simulink model "Manipulator_Dynamics_testing"  (R2019b)
settings: Solver=ode1  StartTime=0.0  StopTime=10  FixedStep=1e-3  RelTol=1e-3  AbsTol=1e-3
InitFcn:
  | parameters
values from neighbouring files (symbols this model uses):
  a = 140/1000    (= 0.14)    [parameters.m]
  d = 23/2000    (= 0.0115)    [parameters.m]
  eta = 0.39    [parameters.m]
  g = 9.81    [parameters.m]
  l_link = a-2*d    (= 0.117)    [parameters.m]
  m = 0.2    [parameters.m]
  mu_cable = 0.17    [parameters.m]
  r = 20.5/1000    (= 0.0205)    [parameters.m]
  r_drum = 0.042    [parameters.m]
libraries: simulink x27, dspindex x18, dspinverses x1
(part 1 of 5)
settings Model: Creator=arund  LastModifiedBy=arund
settings SolverCC: MaxConsecutiveMinStep=10
settings DataIOCC: SaveState=on

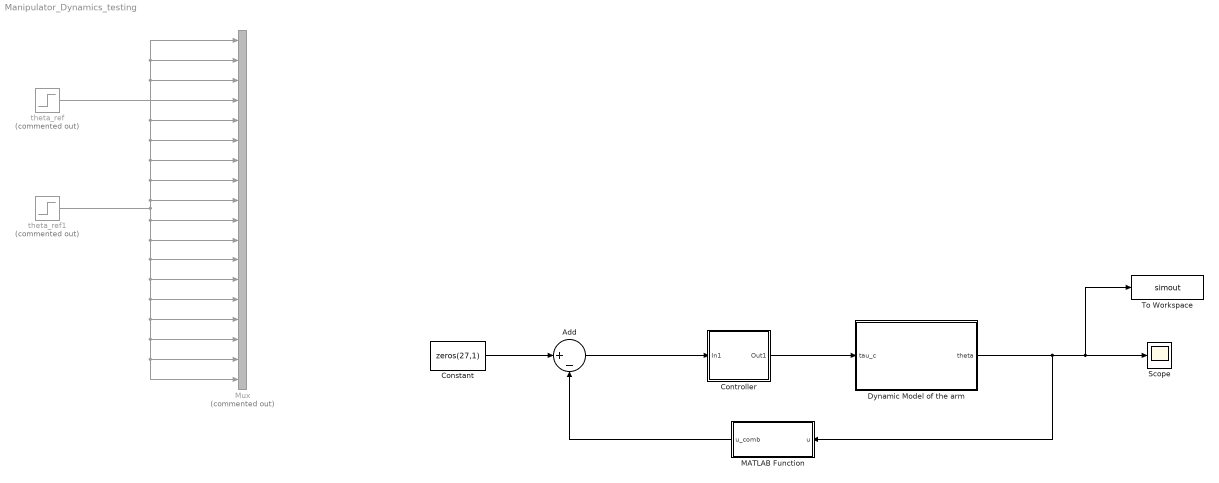
== system Manipulator_Dynamics_testing ==
  Add : Sum  Inputs=|+-
  Constant : Constant  Value=zeros(27,1)
  Controller : Subsystem
  Dynamic Model of the arm : Subsystem
  MATLAB Function : MATLAB Function  TreatAsAtomicUnit=on
  Mux : Mux  Commented=on  Inputs=18
  Scope : Scope
  To Workspace : ToWorkspace  VariableName=simout  SampleTime=-1
  theta_ref : Step  Commented=on  SampleTime=0
  theta_ref1 : Step  Commented=on  After=0  SampleTime=0
  wires:
  Dynamic Model of the arm/1(theta) -> To Workspace/1, Scope/1, MATLAB Function/1(u)
  theta_ref/1 -> Mux/4
  theta_ref1/1 -> Mux/6, Mux/5, Mux/3, Mux/2, Mux/1, Mux/7, Mux/8, Mux/9, Mux/14, Mux/15, Mux/16, Mux/17, Mux/18, Mux/13, Mux/12, Mux/11, Mux/10
  Constant/1 -> Add/1
  MATLAB Function/1(u_comb) -> Add/2
  Add/1 -> Controller/1(In1)
  Controller/1(Out1) -> Dynamic Model of the arm/1(tau_c)

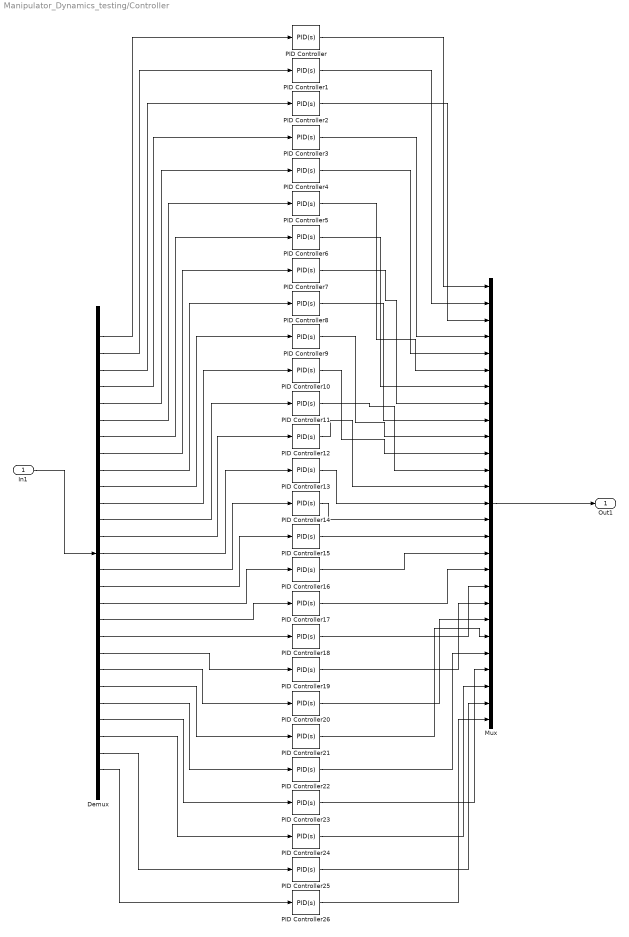
== system Manipulator_Dynamics_testing/Controller ==
  In1 : Inport
  Demux : Demux  Outputs=27
  Mux : Mux  Inputs=27
  PID Controller{,1..23} (24 alike) : simulink/Continuous/PID Controller  Controller=PID  Form=Parallel  TimeDomain=Continuous-time  SampleTime=-1  IntegratorMethod=Forward Euler  FilterMethod=Forward Euler  ControllerParametersSource=internal  P=0  I=0  D=0  UseFilter=on  N=100  TunerSelectOption=Transfer Function Based (PID Tuner App)  InitialConditionSource=internal  InitialConditionForIntegrator=0  InitialConditionForFilter=0  DifferentiatorICPrevScaledInput=0  ExternalReset=none  TrackingMode=off  Kt=1  LimitOutput=off  UpperSaturationLimit=inf  LowerSaturationLimit=-inf  LinearizeAsGain=on  AntiWindupMode=none  Kb=1  POutMin=[]  POutMax=[]  IOutMin=[]  IOutMax=[]  DOutMin=[]  DOutMax=[]  NOutMin=[]  NOutMax=[]  SumOutMin=[]  SumOutMax=[]  SaturationOutMin=[]  SaturationOutMax=[]  PParamMin=[]  PParamMax=[]  IParamMin=[]  IParamMax=[]  DParamMin=[]  DParamMax=[]  NParamMin=[]  NParamMax=[]  KbParamMin=[]  KbParamMax=[]  KtParamMin=[]  KtParamMax=[]  KbOutMin=[]  KbOutMax=[]  KtOutMin=[]  KtOutMax=[]  IntegratorOutMin=[]  IntegratorOutMax=[]  FilterOutMin=[]  FilterOutMax=[]  SumI1OutMin=[]  SumI1OutMax=[]  SumI2OutMin=[]  SumI2OutMax=[]  SumI3OutMin=[]  SumI3OutMax=[]  SumI4OutMin=[]  SumI4OutMax=[]  SumDOutMin=[]  SumDOutMax=[]  DifferentiatorOutMin=[]  DifferentiatorOutMax=[]  FilterDiffOutCoefMin=[]  FilterDiffOutCoefMax=[]  ReciprocalOutMin=[]  ReciprocalOutMax=[]  SumDenOutMin=[]  SumDenOutMax=[]  SumNumOutMin=[]  SumNumOutMax=[]  DivideOutMin=[]  DivideOutMax=[]  IntegratorContinuousStateAttributes=''  IntegratorStateMustResolveToSignalObject=off  IntegratorRTWStateStorageClass=Auto  FilterContinuousStateAttributes=''  FilterStateMustResolveToSignalObject=off  FilterRTWStateStorageClass=Auto  ParallelPVariant=InternalParameters  IdealPVariant=Disabled  IVariant=InternalParameters  DVariant=InternalParameters  IntegratorVariant=Continuous  SatVariant=Disabled  AWVariant=Passthrough  PCopyVariant=Disabled  TRVariant=Disabled  FdbkBlocksVariant=Forward  IdealPFdbkVariant=Disabled  SatFdbkVariant=Disabled  DerivativeFilterVariant=ContFilter  NVariant=InternalParameters  NCopyVariant=Disabled  FilterICVariant=InternalICsFilter  IntegratorICVariant=InternalICs  ExternalResetVariant=Disabled  TRSumVariant=Passthrough  SumFdbkVariant=Disabled  SumVariant=Sum_PID
  PID Controller24 : simulink/Continuous/PID Controller  Controller=PID  Form=Parallel  TimeDomain=Continuous-time  SampleTime=-1  IntegratorMethod=Forward Euler  FilterMethod=Forward Euler  ControllerParametersSource=internal  P=10  I=0  D=10  UseFilter=on  N=100  TunerSelectOption=Transfer Function Based (PID Tuner App)  InitialConditionSource=internal  InitialConditionForIntegrator=0  InitialConditionForFilter=0  DifferentiatorICPrevScaledInput=0  ExternalReset=none  TrackingMode=off  Kt=1  LimitOutput=off  UpperSaturationLimit=inf  LowerSaturationLimit=-inf  LinearizeAsGain=on  AntiWindupMode=none  Kb=1  POutMin=[]  POutMax=[]  IOutMin=[]  IOutMax=[]  DOutMin=[]  DOutMax=[]  NOutMin=[]  NOutMax=[]  SumOutMin=[]  SumOutMax=[]  SaturationOutMin=[]  SaturationOutMax=[]  PParamMin=[]  PParamMax=[]  IParamMin=[]  IParamMax=[]  DParamMin=[]  DParamMax=[]  NParamMin=[]  NParamMax=[]  KbParamMin=[]  KbParamMax=[]  KtParamMin=[]  KtParamMax=[]  KbOutMin=[]  KbOutMax=[]  KtOutMin=[]  KtOutMax=[]  IntegratorOutMin=[]  IntegratorOutMax=[]  FilterOutMin=[]  FilterOutMax=[]  SumI1OutMin=[]  SumI1OutMax=[]  SumI2OutMin=[]  SumI2OutMax=[]  SumI3OutMin=[]  SumI3OutMax=[]  SumI4OutMin=[]  SumI4OutMax=[]  SumDOutMin=[]  SumDOutMax=[]  DifferentiatorOutMin=[]  DifferentiatorOutMax=[]  FilterDiffOutCoefMin=[]  FilterDiffOutCoefMax=[]  ReciprocalOutMin=[]  ReciprocalOutMax=[]  SumDenOutMin=[]  SumDenOutMax=[]  SumNumOutMin=[]  SumNumOutMax=[]  DivideOutMin=[]  DivideOutMax=[]  IntegratorContinuousStateAttributes=''  IntegratorStateMustResolveToSignalObject=off  IntegratorRTWStateStorageClass=Auto  FilterContinuousStateAttributes=''  FilterStateMustResolveToSignalObject=off  FilterRTWStateStorageClass=Auto  ParallelPVariant=InternalParameters  IdealPVariant=Disabled  IVariant=InternalParameters  DVariant=InternalParameters  IntegratorVariant=Continuous  SatVariant=Disabled  AWVariant=Passthrough  PCopyVariant=Disabled  TRVariant=Disabled  FdbkBlocksVariant=Forward  IdealPFdbkVariant=Disabled  SatFdbkVariant=Disabled  DerivativeFilterVariant=ContFilter  NVariant=InternalParameters  NCopyVariant=Disabled  FilterICVariant=InternalICsFilter  IntegratorICVariant=InternalICs  ExternalResetVariant=Disabled  TRSumVariant=Passthrough  SumFdbkVariant=Disabled  SumVariant=Sum_PID
  PID Controller25 : simulink/Continuous/PID Controller  Controller=PID  Form=Parallel  TimeDomain=Continuous-time  SampleTime=-1  IntegratorMethod=Forward Euler  FilterMethod=Forward Euler  ControllerParametersSource=internal  P=10  I=0  D=10  UseFilter=on  N=100  TunerSelectOption=Transfer Function Based (PID Tuner App)  InitialConditionSource=internal  InitialConditionForIntegrator=0  InitialConditionForFilter=0  DifferentiatorICPrevScaledInput=0  ExternalReset=none  TrackingMode=off  Kt=1  LimitOutput=off  UpperSaturationLimit=inf  LowerSaturationLimit=-inf  LinearizeAsGain=on  AntiWindupMode=none  Kb=1  POutMin=[]  POutMax=[]  IOutMin=[]  IOutMax=[]  DOutMin=[]  DOutMax=[]  NOutMin=[]  NOutMax=[]  SumOutMin=[]  SumOutMax=[]  SaturationOutMin=[]  SaturationOutMax=[]  PParamMin=[]  PParamMax=[]  IParamMin=[]  IParamMax=[]  DParamMin=[]  DParamMax=[]  NParamMin=[]  NParamMax=[]  KbParamMin=[]  KbParamMax=[]  KtParamMin=[]  KtParamMax=[]  KbOutMin=[]  KbOutMax=[]  KtOutMin=[]  KtOutMax=[]  IntegratorOutMin=[]  IntegratorOutMax=[]  FilterOutMin=[]  FilterOutMax=[]  SumI1OutMin=[]  SumI1OutMax=[]  SumI2OutMin=[]  SumI2OutMax=[]  SumI3OutMin=[]  SumI3OutMax=[]  SumI4OutMin=[]  SumI4OutMax=[]  SumDOutMin=[]  SumDOutMax=[]  DifferentiatorOutMin=[]  DifferentiatorOutMax=[]  FilterDiffOutCoefMin=[]  FilterDiffOutCoefMax=[]  ReciprocalOutMin=[]  ReciprocalOutMax=[]  SumDenOutMin=[]  SumDenOutMax=[]  SumNumOutMin=[]  SumNumOutMax=[]  DivideOutMin=[]  DivideOutMax=[]  IntegratorContinuousStateAttributes=''  IntegratorStateMustResolveToSignalObject=off  IntegratorRTWStateStorageClass=Auto  FilterContinuousStateAttributes=''  FilterStateMustResolveToSignalObject=off  FilterRTWStateStorageClass=Auto  ParallelPVariant=InternalParameters  IdealPVariant=Disabled  IVariant=InternalParameters  DVariant=InternalParameters  IntegratorVariant=Continuous  SatVariant=Disabled  AWVariant=Passthrough  PCopyVariant=Disabled  TRVariant=Disabled  FdbkBlocksVariant=Forward  IdealPFdbkVariant=Disabled  SatFdbkVariant=Disabled  DerivativeFilterVariant=ContFilter  NVariant=InternalParameters  NCopyVariant=Disabled  FilterICVariant=InternalICsFilter  IntegratorICVariant=InternalICs  ExternalResetVariant=Disabled  TRSumVariant=Passthrough  SumFdbkVariant=Disabled  SumVariant=Sum_PID
  PID Controller26 : simulink/Continuous/PID Controller  Controller=PID  Form=Parallel  TimeDomain=Continuous-time  SampleTime=-1  IntegratorMethod=Forward Euler  FilterMethod=Forward Euler  ControllerParametersSource=internal  P=10  I=0  D=10  UseFilter=on  N=100  TunerSelectOption=Transfer Function Based (PID Tuner App)  InitialConditionSource=internal  InitialConditionForIntegrator=0  InitialConditionForFilter=0  DifferentiatorICPrevScaledInput=0  ExternalReset=none  TrackingMode=off  Kt=1  LimitOutput=off  UpperSaturationLimit=inf  LowerSaturationLimit=-inf  LinearizeAsGain=on  AntiWindupMode=none  Kb=1  POutMin=[]  POutMax=[]  IOutMin=[]  IOutMax=[]  DOutMin=[]  DOutMax=[]  NOutMin=[]  NOutMax=[]  SumOutMin=[]  SumOutMax=[]  SaturationOutMin=[]  SaturationOutMax=[]  PParamMin=[]  PParamMax=[]  IParamMin=[]  IParamMax=[]  DParamMin=[]  DParamMax=[]  NParamMin=[]  NParamMax=[]  KbParamMin=[]  KbParamMax=[]  KtParamMin=[]  KtParamMax=[]  KbOutMin=[]  KbOutMax=[]  KtOutMin=[]  KtOutMax=[]  IntegratorOutMin=[]  IntegratorOutMax=[]  FilterOutMin=[]  FilterOutMax=[]  SumI1OutMin=[]  SumI1OutMax=[]  SumI2OutMin=[]  SumI2OutMax=[]  SumI3OutMin=[]  SumI3OutMax=[]  SumI4OutMin=[]  SumI4OutMax=[]  SumDOutMin=[]  SumDOutMax=[]  DifferentiatorOutMin=[]  DifferentiatorOutMax=[]  FilterDiffOutCoefMin=[]  FilterDiffOutCoefMax=[]  ReciprocalOutMin=[]  ReciprocalOutMax=[]  SumDenOutMin=[]  SumDenOutMax=[]  SumNumOutMin=[]  SumNumOutMax=[]  DivideOutMin=[]  DivideOutMax=[]  IntegratorContinuousStateAttributes=''  IntegratorStateMustResolveToSignalObject=off  IntegratorRTWStateStorageClass=Auto  FilterContinuousStateAttributes=''  FilterStateMustResolveToSignalObject=off  FilterRTWStateStorageClass=Auto  ParallelPVariant=InternalParameters  IdealPVariant=Disabled  IVariant=InternalParameters  DVariant=InternalParameters  IntegratorVariant=Continuous  SatVariant=Disabled  AWVariant=Passthrough  PCopyVariant=Disabled  TRVariant=Disabled  FdbkBlocksVariant=Forward  IdealPFdbkVariant=Disabled  SatFdbkVariant=Disabled  DerivativeFilterVariant=ContFilter  NVariant=InternalParameters  NCopyVariant=Disabled  FilterICVariant=InternalICsFilter  IntegratorICVariant=InternalICs  ExternalResetVariant=Disabled  TRSumVariant=Passthrough  SumFdbkVariant=Disabled  SumVariant=Sum_PID
  Out1 : Outport
  wires:
  In1/1 -> Demux/1
  Mux/1 -> Out1/1
  PID Controller/1 -> Mux/1
  PID Controller1/1 -> Mux/2
  PID Controller2/1 -> Mux/3
  PID Controller3/1 -> Mux/4
  PID Controller4/1 -> Mux/5
  PID Controller5/1 -> Mux/6
  PID Controller6/1 -> Mux/7
  PID Controller7/1 -> Mux/8
  PID Controller8/1 -> Mux/9
  PID Controller9/1 -> Mux/10
  PID Controller10/1 -> Mux/11
  PID Controller11/1 -> Mux/12
  PID Controller12/1 -> Mux/13
  PID Controller13/1 -> Mux/14
  PID Controller14/1 -> Mux/15
  PID Controller15/1 -> Mux/16
  PID Controller16/1 -> Mux/17
  PID Controller17/1 -> Mux/18
  PID Controller18/1 -> Mux/19
  PID Controller19/1 -> Mux/20
  PID Controller20/1 -> Mux/21
  PID Controller21/1 -> Mux/22
  PID Controller22/1 -> Mux/23
  PID Controller23/1 -> Mux/24
  PID Controller24/1 -> Mux/25
  PID Controller25/1 -> Mux/26
  PID Controller26/1 -> Mux/27
  Demux/1 -> PID Controller/1
  Demux/2 -> PID Controller1/1
  Demux/3 -> PID Controller2/1
  Demux/4 -> PID Controller3/1
  Demux/5 -> PID Controller4/1
  Demux/6 -> PID Controller5/1
  Demux/7 -> PID Controller6/1
  Demux/8 -> PID Controller7/1
  Demux/9 -> PID Controller8/1
  Demux/10 -> PID Controller9/1
  Demux/11 -> PID Controller10/1
  Demux/12 -> PID Controller11/1
  Demux/13 -> PID Controller12/1
  Demux/14 -> PID Controller13/1
  Demux/15 -> PID Controller14/1
  Demux/16 -> PID Controller15/1
  Demux/17 -> PID Controller16/1
  Demux/18 -> PID Controller17/1
  Demux/19 -> PID Controller18/1
  Demux/20 -> PID Controller19/1
  Demux/21 -> PID Controller20/1
  Demux/22 -> PID Controller21/1
  Demux/23 -> PID Controller22/1
  Demux/24 -> PID Controller23/1
  Demux/25 -> PID Controller24/1
  Demux/26 -> PID Controller25/1
  Demux/27 -> PID Controller26/1

== system Manipulator_Dynamics_testing/Dynamic Model of the arm ==
  tau_c : Inport
  Integrator : Integrator
  M_inv(theta) : Subsystem
  Matrix Multiply : Product  Multiplication=Matrix(*)
  Subsystem : Subsystem
  h(theta,d_theta) : Subsystem
  theta : Outport
  wires:
  Integrator/1 -> Subsystem/1(d_theta), h(theta,d_theta)/2(d_theta)  "d_theta"
  Matrix Multiply/1 -> Integrator/1  "dd_theta"
  M_inv(theta)/1(M_inv) -> Matrix Multiply/1
  tau_c/1 -> h(theta,d_theta)/3(tau_c), M_inv(theta)/2(tau_c)
  h(theta,d_theta)/1(h) -> Matrix Multiply/2
  Subsystem/1(Out1) -> M_inv(theta)/1(theta), h(theta,d_theta)/1(theta), theta/1

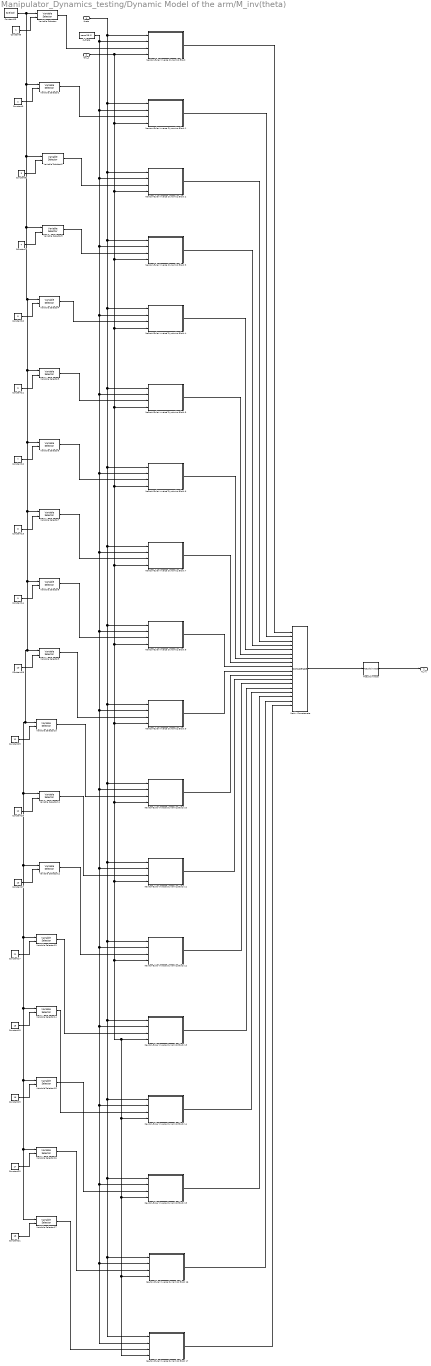
== system Manipulator_Dynamics_testing/Dynamic Model of the arm/M_inv(theta) ==
  theta : Inport
  tau_c : Inport  Port=2
  Constant10 : Constant  Value=5
  Constant11 : Constant  Value=6
  Constant12 : Constant  Value=7
  Constant13 : Constant  Value=8
  Constant14 : Constant  Value=9
  Constant15 : Constant  Value=eye(18)
  Constant17 : Constant  Value=14
  Constant18 : Constant  Value=15
  Constant19 : Constant  Value=16
  Constant20 : Constant  Value=17
  Constant21 : Constant  Value=18
  Constant26 : Constant  Value=12
  Constant27 : Constant  Value=13
  Constant28 : Constant  Value=10
  Constant29 : Constant  Value=11
  Constant6 : Constant  Value=3
  Constant7 : Constant  Value=4
  Constant8 : Constant
  Constant9 : Constant  Value=2
  Matrix Concatenate : Concatenate  NumInputs=18  Mode=Multidimensional array  ConcatenateDimension=2
  "Newton-Euler Inverse Dynamics Block " : Subsystem
  Newton-Euler Inverse Dynamics Block 1 : Subsystem
  Newton-Euler Inverse Dynamics Block 10 : Subsystem
  Newton-Euler Inverse Dynamics Block 11 : Subsystem
  Newton-Euler Inverse Dynamics Block 12 : Subsystem
  Newton-Euler Inverse Dynamics Block 13 : Subsystem
  Newton-Euler Inverse Dynamics Block 14 : Subsystem
  Newton-Euler Inverse Dynamics Block 15 : Subsystem
  Newton-Euler Inverse Dynamics Block 16 : Subsystem
  Newton-Euler Inverse Dynamics Block 17 : Subsystem
  Newton-Euler Inverse Dynamics Block 2 : Subsystem
  Newton-Euler Inverse Dynamics Block 3 : Subsystem
  Newton-Euler Inverse Dynamics Block 4 : Subsystem
  Newton-Euler Inverse Dynamics Block 5 : Subsystem
  Newton-Euler Inverse Dynamics Block 6 : Subsystem
  Newton-Euler Inverse Dynamics Block 7 : Subsystem
  Newton-Euler Inverse Dynamics Block 8 : Subsystem
  Newton-Euler Inverse Dynamics Block 9 : Subsystem
  Pseudoinverse : dspinverses/Pseudoinverse  wanterr=off  SimulateUsing=Interpreted execution
      settings: SourceProductName=DSP System Toolbox  SourceProductBaseCode=DS
  Variable Selector{,1..17} (18 alike) : dspindex/Variable Selector  NumInputs=1  rowsOrCols=Columns  IdxMode=Variable  Elements=[1 3]  ZerOneIdxMode=One-based  errmode=Clip Index  FillMode=on  FillValues=0
  d_theta : Constant  Value=zeros(18,1)
  M_inv : Outport
  wires:
  Variable Selector/1 -> "Newton-Euler Inverse Dynamics Block "/3(dd_theta)
  Constant8/1 -> Variable Selector/2
  Variable Selector1/1 -> Newton-Euler Inverse Dynamics Block 1/3(dd_theta)
  Constant9/1 -> Variable Selector1/2
  Matrix Concatenate/1 -> Pseudoinverse/1
  Constant6/1 -> Variable Selector2/2
  Variable Selector2/1 -> Newton-Euler Inverse Dynamics Block 2/3(dd_theta)
  Constant7/1 -> Variable Selector3/2
  Variable Selector3/1 -> Newton-Euler Inverse Dynamics Block 3/3(dd_theta)
  Constant10/1 -> Variable Selector4/2
  Variable Selector4/1 -> Newton-Euler Inverse Dynamics Block 4/3(dd_theta)
  Constant11/1 -> Variable Selector5/2
  Variable Selector5/1 -> Newton-Euler Inverse Dynamics Block 5/3(dd_theta)
  Constant12/1 -> Variable Selector6/2
  Variable Selector6/1 -> Newton-Euler Inverse Dynamics Block 6/3(dd_theta)
  Constant13/1 -> Variable Selector7/2
  Variable Selector7/1 -> Newton-Euler Inverse Dynamics Block 7/3(dd_theta)
  Constant14/1 -> Variable Selector8/2
  Variable Selector8/1 -> Newton-Euler Inverse Dynamics Block 8/3(dd_theta)
  Pseudoinverse/1 -> M_inv/1
  Variable Selector11/1 -> Newton-Euler Inverse Dynamics Block 11/3(dd_theta)
  Constant26/1 -> Variable Selector11/2
  Variable Selector14/1 -> Newton-Euler Inverse Dynamics Block 14/3(dd_theta)
  Constant18/1 -> Variable Selector14/2
  Variable Selector17/1 -> Newton-Euler Inverse Dynamics Block 17/3(dd_theta)
  Constant21/1 -> Variable Selector17/2
  Constant15/1 -> Variable Selector9/1, Variable Selector10/1, Variable Selector17/1, Variable Selector16/1, Variable Selector15/1, Variable Selector14/1, Variable Selector13/1, Variable Selector12/1, Variable Selector11/1, Variable Selector8/1, Variable Selector7/1, Variable Selector6/1, Variable Selector5/1, Variable Selector4/1, Variable Selector3/1, Variable Selector2/1, Variable Selector1/1, Variable Selector/1
  d_theta/1 -> "Newton-Euler Inverse Dynamics Block "/2(d_theta), Newton-Euler Inverse Dynamics Block 6/2(d_theta), Newton-Euler Inverse Dynamics Block 7/2(d_theta), Newton-Euler Inverse Dynamics Block 8/2(d_theta), Newton-Euler Inverse Dynamics Block 9/2(d_theta), Newton-Euler Inverse Dynamics Block 11/2(d_theta), Newton-Euler Inverse Dynamics Block 12/2(d_theta), Newton-Euler Inverse Dynamics Block 17/2(d_theta), Newton-Euler Inverse Dynamics Block 16/2(d_theta), Newton-Euler Inverse Dynamics Block 15/2(d_theta), Newton-Euler Inverse Dynamics Block 14/2(d_theta), Newton-Euler Inverse Dynamics Block 13/2(d_theta), Newton-Euler Inverse Dynamics Block 10/2(d_theta), Newton-Euler Inverse Dynamics Block 5/2(d_theta), Newton-Euler Inverse Dynamics Block 4/2(d_theta), Newton-Euler Inverse Dynamics Block 3/2(d_theta), Newton-Euler Inverse Dynamics Block 2/2(d_theta), Newton-Euler Inverse Dynamics Block 1/2(d_theta)
  theta/1 -> "Newton-Euler Inverse Dynamics Block "/1(theta), Newton-Euler Inverse Dynamics Block 1/1(theta), Newton-Euler Inverse Dynamics Block 3/1(theta), Newton-Euler Inverse Dynamics Block 4/1(theta), Newton-Euler Inverse Dynamics Block 5/1(theta), Newton-Euler Inverse Dynamics Block 6/1(theta), Newton-Euler Inverse Dynamics Block 7/1(theta), Newton-Euler Inverse Dynamics Block 8/1(theta), Newton-Euler Inverse Dynamics Block 9/1(theta), Newton-Euler Inverse Dynamics Block 10/1(theta), Newton-Euler Inverse Dynamics Block 11/1(theta), Newton-Euler Inverse Dynamics Block 12/1(theta), Newton-Euler Inverse Dynamics Block 13/1(theta), Newton-Euler Inverse Dynamics Block 14/1(theta), Newton-Euler Inverse Dynamics Block 16/1(theta), Newton-Euler Inverse Dynamics Block 17/1(theta), Newton-Euler Inverse Dynamics Block 15/1(theta), Newton-Euler Inverse Dynamics Block 2/1(theta)
  Constant28/1 -> Variable Selector9/2
  Variable Selector13/1 -> Newton-Euler Inverse Dynamics Block 13/3(dd_theta)
  Constant17/1 -> Variable Selector13/2
  Constant20/1 -> Variable Selector16/2
  Constant19/1 -> Variable Selector15/2
  Constant29/1 -> Variable Selector10/2
  Variable Selector10/1 -> Newton-Euler Inverse Dynamics Block 10/3(dd_theta)
  Variable Selector9/1 -> Newton-Euler Inverse Dynamics Block 9/3(dd_theta)
  Constant27/1 -> Variable Selector12/2
  Variable Selector12/1 -> Newton-Euler Inverse Dynamics Block 12/3(dd_theta)
  Variable Selector15/1 -> Newton-Euler Inverse Dynamics Block 15/3(dd_theta)
  Variable Selector16/1 -> Newton-Euler Inverse Dynamics Block 16/3(dd_theta)
  tau_c/1 -> Newton-Euler Inverse Dynamics Block 6/4(tau_c), Newton-Euler Inverse Dynamics Block 11/4(tau_c), Newton-Euler Inverse Dynamics Block 12/4(tau_c), Newton-Euler Inverse Dynamics Block 13/4(tau_c), Newton-Euler Inverse Dynamics Block 14/4(tau_c), Newton-Euler Inverse Dynamics Block 15/4(tau_c), Newton-Euler Inverse Dynamics Block 17/4(tau_c), Newton-Euler Inverse Dynamics Block 16/4(tau_c), Newton-Euler Inverse Dynamics Block 10/4(tau_c), Newton-Euler Inverse Dynamics Block 9/4(tau_c), Newton-Euler Inverse Dynamics Block 8/4(tau_c), Newton-Euler Inverse Dynamics Block 7/4(tau_c), Newton-Euler Inverse Dynamics Block 5/4(tau_c), Newton-Euler Inverse Dynamics Block 4/4(tau_c), Newton-Euler Inverse Dynamics Block 3/4(tau_c), Newton-Euler Inverse Dynamics Block 2/4(tau_c), Newton-Euler Inverse Dynamics Block 1/4(tau_c), "Newton-Euler Inverse Dynamics Block "/4(tau_c)
  "Newton-Euler Inverse Dynamics Block "/1(tau) -> Matrix Concatenate/1
  Newton-Euler Inverse Dynamics Block 1/1(tau) -> Matrix Concatenate/2
  Newton-Euler Inverse Dynamics Block 2/1(tau) -> Matrix Concatenate/3
  Newton-Euler Inverse Dynamics Block 3/1(tau) -> Matrix Concatenate/4
  Newton-Euler Inverse Dynamics Block 4/1(tau) -> Matrix Concatenate/5
  Newton-Euler Inverse Dynamics Block 5/1(tau) -> Matrix Concatenate/6
  Newton-Euler Inverse Dynamics Block 6/1(tau) -> Matrix Concatenate/7
  Newton-Euler Inverse Dynamics Block 7/1(tau) -> Matrix Concatenate/8
  Newton-Euler Inverse Dynamics Block 8/1(tau) -> Matrix Concatenate/9
  Newton-Euler Inverse Dynamics Block 9/1(tau) -> Matrix Concatenate/10
  Newton-Euler Inverse Dynamics Block 10/1(tau) -> Matrix Concatenate/11
  Newton-Euler Inverse Dynamics Block 11/1(tau) -> Matrix Concatenate/12
  Newton-Euler Inverse Dynamics Block 12/1(tau) -> Matrix Concatenate/13
  Newton-Euler Inverse Dynamics Block 13/1(tau) -> Matrix Concatenate/14
  Newton-Euler Inverse Dynamics Block 14/1(tau) -> Matrix Concatenate/15
  Newton-Euler Inverse Dynamics Block 15/1(tau) -> Matrix Concatenate/16
  Newton-Euler Inverse Dynamics Block 16/1(tau) -> Matrix Concatenate/17
  Newton-Euler Inverse Dynamics Block 17/1(tau) -> Matrix Concatenate/18

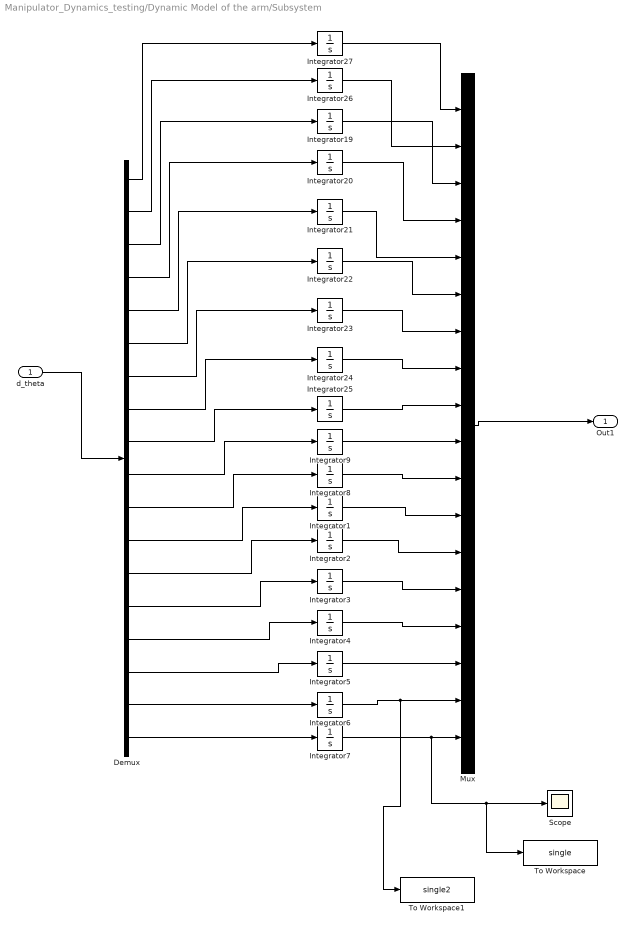
== system Manipulator_Dynamics_testing/Dynamic Model of the arm/Subsystem ==
  d_theta : Inport
  Demux : Demux  Outputs=18
  Integrator{1..6,8..9,19..27} (17 alike) : Integrator
  Integrator7 : Integrator  InitialCondition=0.1
  Mux : Mux  Inputs=18
  Scope : Scope
  To Workspace : ToWorkspace  VariableName=single  SampleTime=-1
  To Workspace1 : ToWorkspace  VariableName=single2  SampleTime=-1
  Out1 : Outport
  wires:
  d_theta/1 -> Demux/1
  Mux/1 -> Out1/1
  Demux/1 -> Integrator27/1
  Demux/2 -> Integrator26/1
  Demux/3 -> Integrator19/1
  Demux/4 -> Integrator20/1
  Demux/5 -> Integrator21/1
  Demux/6 -> Integrator22/1
  Demux/7 -> Integrator23/1
  Demux/8 -> Integrator24/1
  Demux/9 -> Integrator25/1
  Demux/10 -> Integrator9/1
  Demux/11 -> Integrator8/1
  Demux/12 -> Integrator1/1
  Demux/13 -> Integrator2/1
  Demux/14 -> Integrator3/1
  Demux/15 -> Integrator4/1
  Demux/16 -> Integrator5/1
  Demux/17 -> Integrator6/1
  Demux/18 -> Integrator7/1
  Integrator7/1 -> To Workspace/1, Scope/1, Mux/18
  Integrator6/1 -> To Workspace1/1, Mux/17
  Integrator5/1 -> Mux/16
  Integrator4/1 -> Mux/15
  Integrator3/1 -> Mux/14
  Integrator2/1 -> Mux/13
  Integrator1/1 -> Mux/12
  Integrator8/1 -> Mux/11
  Integrator9/1 -> Mux/10
  Integrator25/1 -> Mux/9
  Integrator24/1 -> Mux/8
  Integrator23/1 -> Mux/7
  Integrator22/1 -> Mux/6
  Integrator21/1 -> Mux/5
  Integrator20/1 -> Mux/4
  Integrator19/1 -> Mux/3
  Integrator26/1 -> Mux/2
  Integrator27/1 -> Mux/1

== system Manipulator_Dynamics_testing/Dynamic Model of the arm/h(theta,d_theta) ==
  theta : Inport
  d_theta : Inport  Port=2
  tau_c : Inport  Port=3
  "Newton-Euler Inverse Dynamics Block " : Subsystem
  dd_theta : Constant  Value=zeros(18,1)
  h : Outport
  wires:
  "Newton-Euler Inverse Dynamics Block "/1(tau) -> h/1
  dd_theta/1 -> "Newton-Euler Inverse Dynamics Block "/3(dd_theta)
  d_theta/1 -> "Newton-Euler Inverse Dynamics Block "/2(d_theta)
  theta/1 -> "Newton-Euler Inverse Dynamics Block "/1(theta)
  tau_c/1 -> "Newton-Euler Inverse Dynamics Block "/4(tau_c)

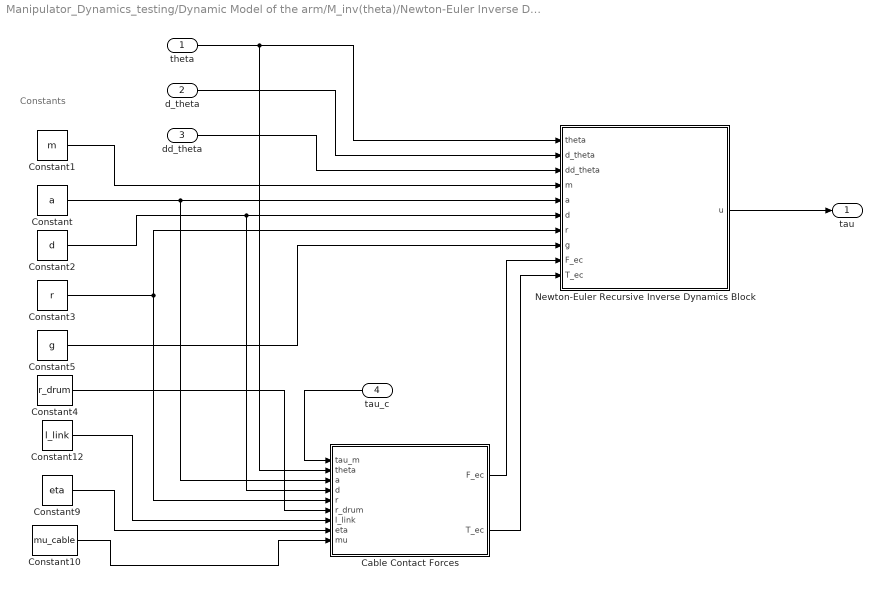
== system Manipulator_Dynamics_testing/Dynamic Model of the arm/M_inv(theta)/Newton-Euler Inverse Dynamics Block  ==
  note: Constants
  theta : Inport
  d_theta : Inport  Port=2
  dd_theta : Inport  Port=3
  tau_c : Inport  Port=4
  Cable Contact Forces : MATLAB Function  TreatAsAtomicUnit=on
  Constant : Constant  Value=a
  Constant1 : Constant  Value=m
  Constant10 : Constant  Value=mu_cable
  Constant12 : Constant  Value=l_link
  Constant2 : Constant  Value=d
  Constant3 : Constant  Value=r
  Constant4 : Constant  Value=r_drum
  Constant5 : Constant  Value=g
  Constant9 : Constant  Value=eta
  Newton-Euler Recursive Inverse Dynamics Block : MATLAB Function  TreatAsAtomicUnit=on
  tau : Outport
  wires:
  Constant/1 -> Cable Contact Forces/3(a), Newton-Euler Recursive Inverse Dynamics Block/5(a)
  dd_theta/1 -> Newton-Euler Recursive Inverse Dynamics Block/3(dd_theta)
  Constant9/1 -> Cable Contact Forces/8(eta)
  Constant4/1 -> Cable Contact Forces/6(r_drum)
  theta/1 -> Newton-Euler Recursive Inverse Dynamics Block/1(theta), Cable Contact Forces/2(theta)
  Constant2/1 -> Cable Contact Forces/4(d), Newton-Euler Recursive Inverse Dynamics Block/6(d)
  Constant3/1 -> Cable Contact Forces/5(r), Newton-Euler Recursive Inverse Dynamics Block/7(r)
  Constant10/1 -> Cable Contact Forces/9(mu)
  d_theta/1 -> Newton-Euler Recursive Inverse Dynamics Block/2(d_theta)
  Constant1/1 -> Newton-Euler Recursive Inverse Dynamics Block/4(m)
  Constant5/1 -> Newton-Euler Recursive Inverse Dynamics Block/8(g)
  Newton-Euler Recursive Inverse Dynamics Block/1(u) -> tau/1
  Cable Contact Forces/2(T_ec) -> Newton-Euler Recursive Inverse Dynamics Block/10(T_ec)
  Cable Contact Forces/1(F_ec) -> Newton-Euler Recursive Inverse Dynamics Block/9(F_ec)
  Constant12/1 -> Cable Contact Forces/7(l_link)
  tau_c/1 -> Cable Contact Forces/1(tau_m)

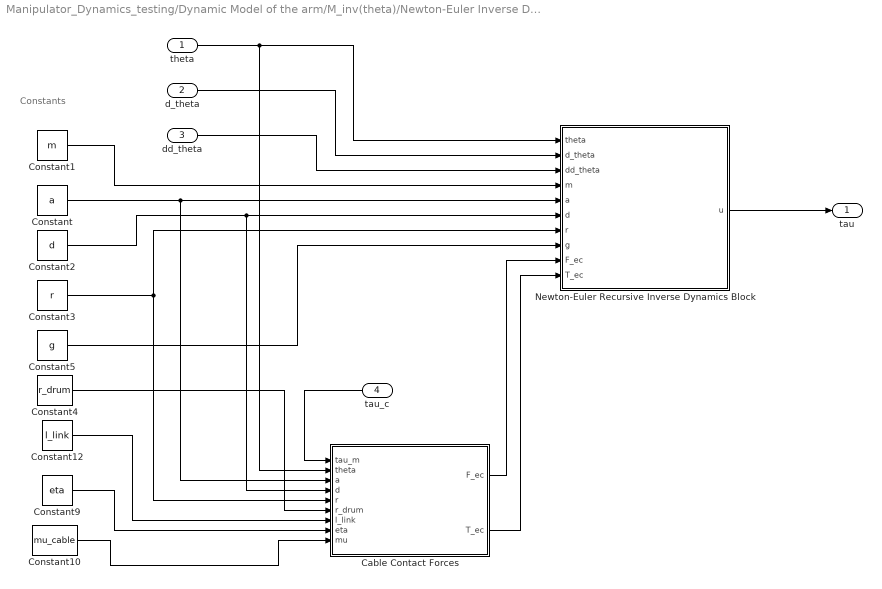
== system Manipulator_Dynamics_testing/Dynamic Model of the arm/M_inv(theta)/Newton-Euler Inverse Dynamics Block 1 ==
  note: Constants
  theta : Inport
  d_theta : Inport  Port=2
  dd_theta : Inport  Port=3
  tau_c : Inport  Port=4
  Cable Contact Forces : MATLAB Function  TreatAsAtomicUnit=on
  Constant : Constant  Value=a
  Constant1 : Constant  Value=m
  Constant10 : Constant  Value=mu_cable
  Constant12 : Constant  Value=l_link
  Constant2 : Constant  Value=d
  Constant3 : Constant  Value=r
  Constant4 : Constant  Value=r_drum
  Constant5 : Constant  Value=g
  Constant9 : Constant  Value=eta
  Newton-Euler Recursive Inverse Dynamics Block : MATLAB Function  TreatAsAtomicUnit=on
  tau : Outport
  wires:
  Constant/1 -> Cable Contact Forces/3(a), Newton-Euler Recursive Inverse Dynamics Block/5(a)
  dd_theta/1 -> Newton-Euler Recursive Inverse Dynamics Block/3(dd_theta)
  Constant9/1 -> Cable Contact Forces/8(eta)
  Constant4/1 -> Cable Contact Forces/6(r_drum)
  theta/1 -> Newton-Euler Recursive Inverse Dynamics Block/1(theta), Cable Contact Forces/2(theta)
  Constant2/1 -> Cable Contact Forces/4(d), Newton-Euler Recursive Inverse Dynamics Block/6(d)
  Constant3/1 -> Cable Contact Forces/5(r), Newton-Euler Recursive Inverse Dynamics Block/7(r)
  Constant10/1 -> Cable Contact Forces/9(mu)
  d_theta/1 -> Newton-Euler Recursive Inverse Dynamics Block/2(d_theta)
  Constant1/1 -> Newton-Euler Recursive Inverse Dynamics Block/4(m)
  Constant5/1 -> Newton-Euler Recursive Inverse Dynamics Block/8(g)
  Newton-Euler Recursive Inverse Dynamics Block/1(u) -> tau/1
  Cable Contact Forces/2(T_ec) -> Newton-Euler Recursive Inverse Dynamics Block/10(T_ec)
  Cable Contact Forces/1(F_ec) -> Newton-Euler Recursive Inverse Dynamics Block/9(F_ec)
  Constant12/1 -> Cable Contact Forces/7(l_link)
  tau_c/1 -> Cable Contact Forces/1(tau_m)

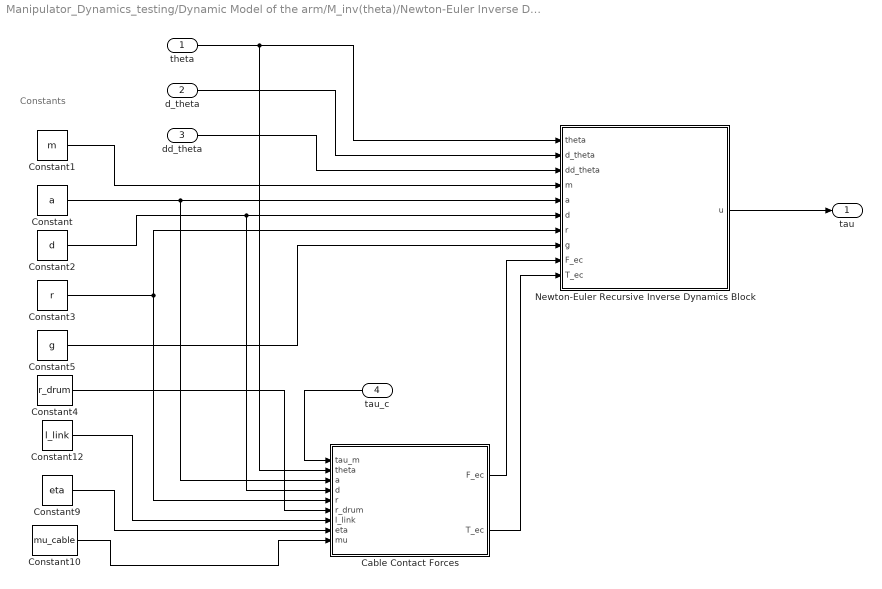
== system Manipulator_Dynamics_testing/Dynamic Model of the arm/M_inv(theta)/Newton-Euler Inverse Dynamics Block 10 ==
  note: Constants
  theta : Inport
  d_theta : Inport  Port=2
  dd_theta : Inport  Port=3
  tau_c : Inport  Port=4
  Cable Contact Forces : MATLAB Function  TreatAsAtomicUnit=on
  Constant : Constant  Value=a
  Constant1 : Constant  Value=m
  Constant10 : Constant  Value=mu_cable
  Constant12 : Constant  Value=l_link
  Constant2 : Constant  Value=d
  Constant3 : Constant  Value=r
  Constant4 : Constant  Value=r_drum
  Constant5 : Constant  Value=g
  Constant9 : Constant  Value=eta
  Newton-Euler Recursive Inverse Dynamics Block : MATLAB Function  TreatAsAtomicUnit=on
  tau : Outport
  wires:
  Constant/1 -> Cable Contact Forces/3(a), Newton-Euler Recursive Inverse Dynamics Block/5(a)
  dd_theta/1 -> Newton-Euler Recursive Inverse Dynamics Block/3(dd_theta)
  Constant9/1 -> Cable Contact Forces/8(eta)
  Constant4/1 -> Cable Contact Forces/6(r_drum)
  theta/1 -> Newton-Euler Recursive Inverse Dynamics Block/1(theta), Cable Contact Forces/2(theta)
  Constant2/1 -> Cable Contact Forces/4(d), Newton-Euler Recursive Inverse Dynamics Block/6(d)
  Constant3/1 -> Cable Contact Forces/5(r), Newton-Euler Recursive Inverse Dynamics Block/7(r)
  Constant10/1 -> Cable Contact Forces/9(mu)
  d_theta/1 -> Newton-Euler Recursive Inverse Dynamics Block/2(d_theta)
  Constant1/1 -> Newton-Euler Recursive Inverse Dynamics Block/4(m)
  Constant5/1 -> Newton-Euler Recursive Inverse Dynamics Block/8(g)
  Newton-Euler Recursive Inverse Dynamics Block/1(u) -> tau/1
  Cable Contact Forces/2(T_ec) -> Newton-Euler Recursive Inverse Dynamics Block/10(T_ec)
  Cable Contact Forces/1(F_ec) -> Newton-Euler Recursive Inverse Dynamics Block/9(F_ec)
  Constant12/1 -> Cable Contact Forces/7(l_link)
  tau_c/1 -> Cable Contact Forces/1(tau_m)

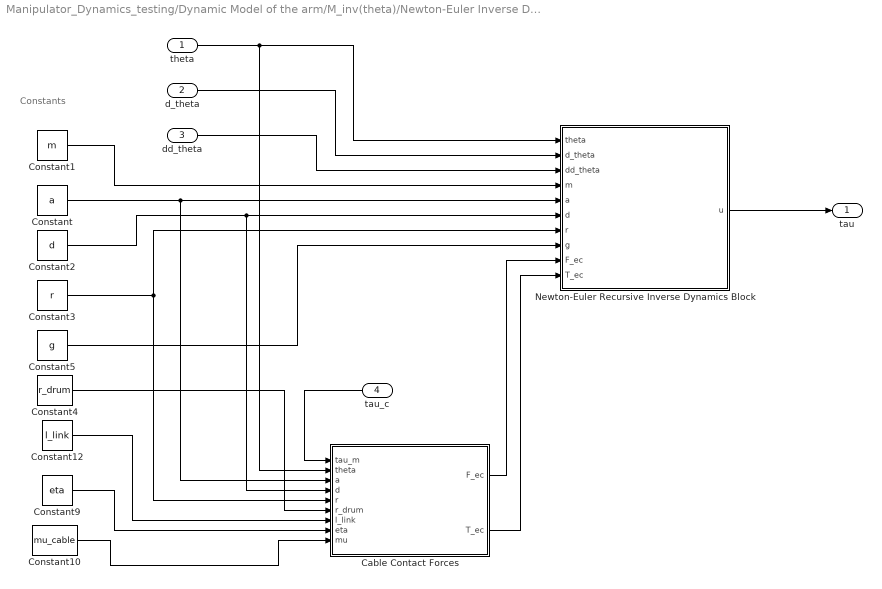
== system Manipulator_Dynamics_testing/Dynamic Model of the arm/M_inv(theta)/Newton-Euler Inverse Dynamics Block 11 ==
  note: Constants
  theta : Inport
  d_theta : Inport  Port=2
  dd_theta : Inport  Port=3
  tau_c : Inport  Port=4
  Cable Contact Forces : MATLAB Function  TreatAsAtomicUnit=on
  Constant : Constant  Value=a
  Constant1 : Constant  Value=m
  Constant10 : Constant  Value=mu_cable
  Constant12 : Constant  Value=l_link
  Constant2 : Constant  Value=d
  Constant3 : Constant  Value=r
  Constant4 : Constant  Value=r_drum
  Constant5 : Constant  Value=g
  Constant9 : Constant  Value=eta
  Newton-Euler Recursive Inverse Dynamics Block : MATLAB Function  TreatAsAtomicUnit=on
  tau : Outport
  wires:
  Constant/1 -> Cable Contact Forces/3(a), Newton-Euler Recursive Inverse Dynamics Block/5(a)
  dd_theta/1 -> Newton-Euler Recursive Inverse Dynamics Block/3(dd_theta)
  Constant9/1 -> Cable Contact Forces/8(eta)
  Constant4/1 -> Cable Contact Forces/6(r_drum)
  theta/1 -> Newton-Euler Recursive Inverse Dynamics Block/1(theta), Cable Contact Forces/2(theta)
  Constant2/1 -> Cable Contact Forces/4(d), Newton-Euler Recursive Inverse Dynamics Block/6(d)
  Constant3/1 -> Cable Contact Forces/5(r), Newton-Euler Recursive Inverse Dynamics Block/7(r)
  Constant10/1 -> Cable Contact Forces/9(mu)
  d_theta/1 -> Newton-Euler Recursive Inverse Dynamics Block/2(d_theta)
  Constant1/1 -> Newton-Euler Recursive Inverse Dynamics Block/4(m)
  Constant5/1 -> Newton-Euler Recursive Inverse Dynamics Block/8(g)
  Newton-Euler Recursive Inverse Dynamics Block/1(u) -> tau/1
  Cable Contact Forces/2(T_ec) -> Newton-Euler Recursive Inverse Dynamics Block/10(T_ec)
  Cable Contact Forces/1(F_ec) -> Newton-Euler Recursive Inverse Dynamics Block/9(F_ec)
  Constant12/1 -> Cable Contact Forces/7(l_link)
  tau_c/1 -> Cable Contact Forces/1(tau_m)

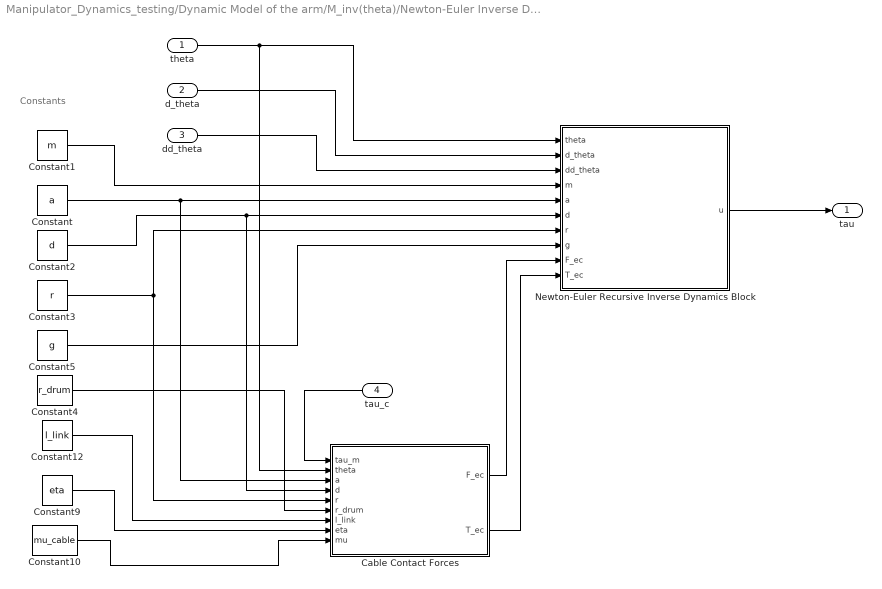
== system Manipulator_Dynamics_testing/Dynamic Model of the arm/M_inv(theta)/Newton-Euler Inverse Dynamics Block 12 ==
  note: Constants
  theta : Inport
  d_theta : Inport  Port=2
  dd_theta : Inport  Port=3
  tau_c : Inport  Port=4
  Cable Contact Forces : MATLAB Function  TreatAsAtomicUnit=on
  Constant : Constant  Value=a
  Constant1 : Constant  Value=m
  Constant10 : Constant  Value=mu_cable
  Constant12 : Constant  Value=l_link
  Constant2 : Constant  Value=d
  Constant3 : Constant  Value=r
  Constant4 : Constant  Value=r_drum
  Constant5 : Constant  Value=g
  Constant9 : Constant  Value=eta
  Newton-Euler Recursive Inverse Dynamics Block : MATLAB Function  TreatAsAtomicUnit=on
  tau : Outport
  wires:
  Constant/1 -> Cable Contact Forces/3(a), Newton-Euler Recursive Inverse Dynamics Block/5(a)
  dd_theta/1 -> Newton-Euler Recursive Inverse Dynamics Block/3(dd_theta)
  Constant9/1 -> Cable Contact Forces/8(eta)
  Constant4/1 -> Cable Contact Forces/6(r_drum)
  theta/1 -> Newton-Euler Recursive Inverse Dynamics Block/1(theta), Cable Contact Forces/2(theta)
  Constant2/1 -> Cable Contact Forces/4(d), Newton-Euler Recursive Inverse Dynamics Block/6(d)
  Constant3/1 -> Cable Contact Forces/5(r), Newton-Euler Recursive Inverse Dynamics Block/7(r)
  Constant10/1 -> Cable Contact Forces/9(mu)
  d_theta/1 -> Newton-Euler Recursive Inverse Dynamics Block/2(d_theta)
  Constant1/1 -> Newton-Euler Recursive Inverse Dynamics Block/4(m)
  Constant5/1 -> Newton-Euler Recursive Inverse Dynamics Block/8(g)
  Newton-Euler Recursive Inverse Dynamics Block/1(u) -> tau/1
  Cable Contact Forces/2(T_ec) -> Newton-Euler Recursive Inverse Dynamics Block/10(T_ec)
  Cable Contact Forces/1(F_ec) -> Newton-Euler Recursive Inverse Dynamics Block/9(F_ec)
  Constant12/1 -> Cable Contact Forces/7(l_link)
  tau_c/1 -> Cable Contact Forces/1(tau_m)

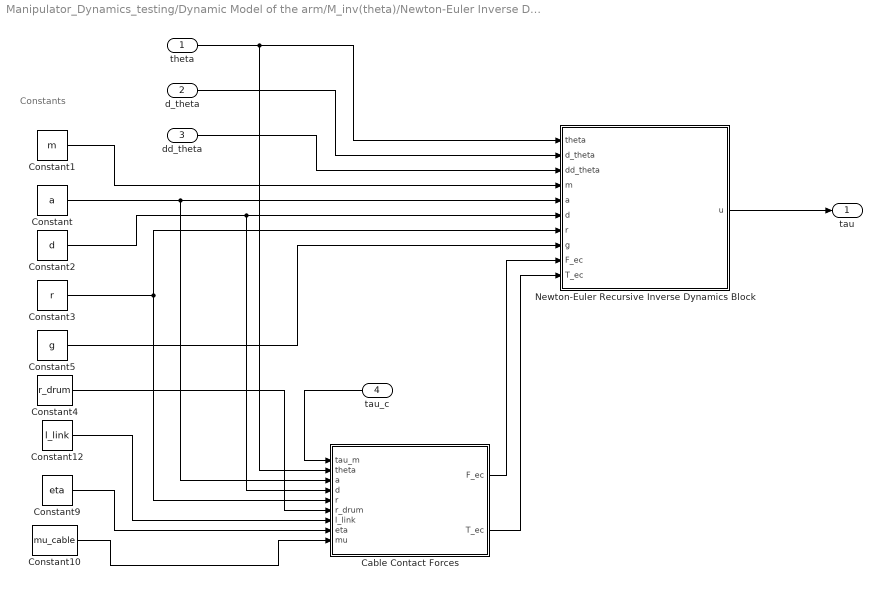
== system Manipulator_Dynamics_testing/Dynamic Model of the arm/M_inv(theta)/Newton-Euler Inverse Dynamics Block 13 ==
  note: Constants
  theta : Inport
  d_theta : Inport  Port=2
  dd_theta : Inport  Port=3
  tau_c : Inport  Port=4
  Cable Contact Forces : MATLAB Function  TreatAsAtomicUnit=on
  Constant : Constant  Value=a
  Constant1 : Constant  Value=m
  Constant10 : Constant  Value=mu_cable
  Constant12 : Constant  Value=l_link
  Constant2 : Constant  Value=d
  Constant3 : Constant  Value=r
  Constant4 : Constant  Value=r_drum
  Constant5 : Constant  Value=g
  Constant9 : Constant  Value=eta
  Newton-Euler Recursive Inverse Dynamics Block : MATLAB Function  TreatAsAtomicUnit=on
  tau : Outport
  wires:
  Constant/1 -> Cable Contact Forces/3(a), Newton-Euler Recursive Inverse Dynamics Block/5(a)
  dd_theta/1 -> Newton-Euler Recursive Inverse Dynamics Block/3(dd_theta)
  Constant9/1 -> Cable Contact Forces/8(eta)
  Constant4/1 -> Cable Contact Forces/6(r_drum)
  theta/1 -> Newton-Euler Recursive Inverse Dynamics Block/1(theta), Cable Contact Forces/2(theta)
  Constant2/1 -> Cable Contact Forces/4(d), Newton-Euler Recursive Inverse Dynamics Block/6(d)
  Constant3/1 -> Cable Contact Forces/5(r), Newton-Euler Recursive Inverse Dynamics Block/7(r)
  Constant10/1 -> Cable Contact Forces/9(mu)
  d_theta/1 -> Newton-Euler Recursive Inverse Dynamics Block/2(d_theta)
  Constant1/1 -> Newton-Euler Recursive Inverse Dynamics Block/4(m)
  Constant5/1 -> Newton-Euler Recursive Inverse Dynamics Block/8(g)
  Newton-Euler Recursive Inverse Dynamics Block/1(u) -> tau/1
  Cable Contact Forces/2(T_ec) -> Newton-Euler Recursive Inverse Dynamics Block/10(T_ec)
  Cable Contact Forces/1(F_ec) -> Newton-Euler Recursive Inverse Dynamics Block/9(F_ec)
  Constant12/1 -> Cable Contact Forces/7(l_link)
  tau_c/1 -> Cable Contact Forces/1(tau_m)

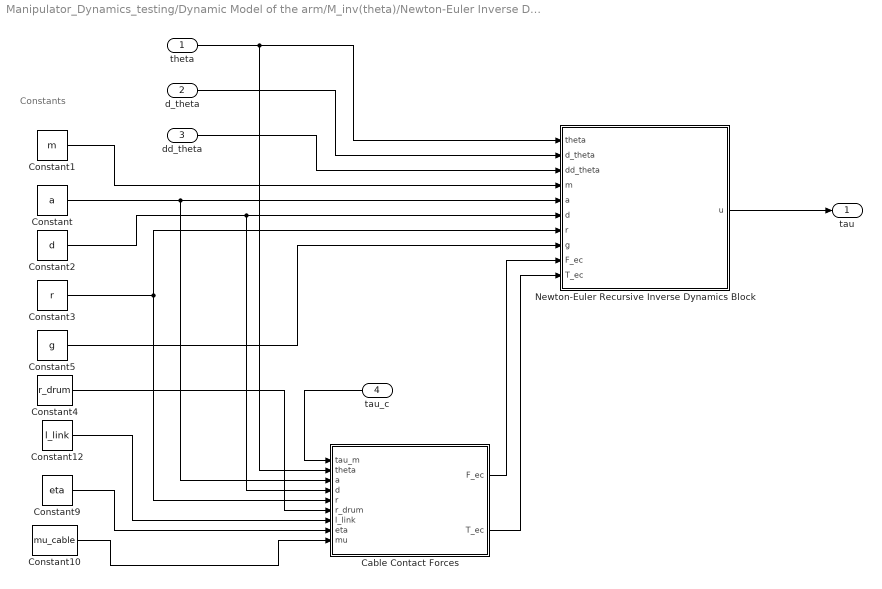
== system Manipulator_Dynamics_testing/Dynamic Model of the arm/M_inv(theta)/Newton-Euler Inverse Dynamics Block 14 ==
  note: Constants
  theta : Inport
  d_theta : Inport  Port=2
  dd_theta : Inport  Port=3
  tau_c : Inport  Port=4
  Cable Contact Forces : MATLAB Function  TreatAsAtomicUnit=on
  Constant : Constant  Value=a
  Constant1 : Constant  Value=m
  Constant10 : Constant  Value=mu_cable
  Constant12 : Constant  Value=l_link
  Constant2 : Constant  Value=d
  Constant3 : Constant  Value=r
  Constant4 : Constant  Value=r_drum
  Constant5 : Constant  Value=g
  Constant9 : Constant  Value=eta
  Newton-Euler Recursive Inverse Dynamics Block : MATLAB Function  TreatAsAtomicUnit=on
  tau : Outport
  wires:
  Constant/1 -> Cable Contact Forces/3(a), Newton-Euler Recursive Inverse Dynamics Block/5(a)
  dd_theta/1 -> Newton-Euler Recursive Inverse Dynamics Block/3(dd_theta)
  Constant9/1 -> Cable Contact Forces/8(eta)
  Constant4/1 -> Cable Contact Forces/6(r_drum)
  theta/1 -> Newton-Euler Recursive Inverse Dynamics Block/1(theta), Cable Contact Forces/2(theta)
  Constant2/1 -> Cable Contact Forces/4(d), Newton-Euler Recursive Inverse Dynamics Block/6(d)
  Constant3/1 -> Cable Contact Forces/5(r), Newton-Euler Recursive Inverse Dynamics Block/7(r)
  Constant10/1 -> Cable Contact Forces/9(mu)
  d_theta/1 -> Newton-Euler Recursive Inverse Dynamics Block/2(d_theta)
  Constant1/1 -> Newton-Euler Recursive Inverse Dynamics Block/4(m)
  Constant5/1 -> Newton-Euler Recursive Inverse Dynamics Block/8(g)
  Newton-Euler Recursive Inverse Dynamics Block/1(u) -> tau/1
  Cable Contact Forces/2(T_ec) -> Newton-Euler Recursive Inverse Dynamics Block/10(T_ec)
  Cable Contact Forces/1(F_ec) -> Newton-Euler Recursive Inverse Dynamics Block/9(F_ec)
  Constant12/1 -> Cable Contact Forces/7(l_link)
  tau_c/1 -> Cable Contact Forces/1(tau_m)

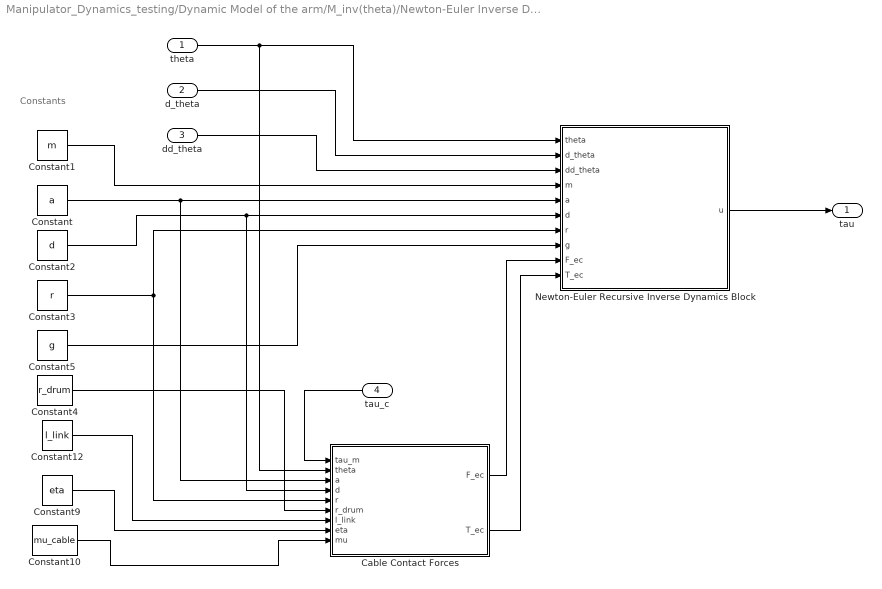
== system Manipulator_Dynamics_testing/Dynamic Model of the arm/M_inv(theta)/Newton-Euler Inverse Dynamics Block 15 ==
  note: Constants
  theta : Inport
  d_theta : Inport  Port=2
  dd_theta : Inport  Port=3
  tau_c : Inport  Port=4
  Cable Contact Forces : MATLAB Function  TreatAsAtomicUnit=on
  Constant : Constant  Value=a
  Constant1 : Constant  Value=m
  Constant10 : Constant  Value=mu_cable
  Constant12 : Constant  Value=l_link
  Constant2 : Constant  Value=d
  Constant3 : Constant  Value=r
  Constant4 : Constant  Value=r_drum
  Constant5 : Constant  Value=g
  Constant9 : Constant  Value=eta
  Newton-Euler Recursive Inverse Dynamics Block : MATLAB Function  TreatAsAtomicUnit=on
  tau : Outport
  wires:
  Constant/1 -> Cable Contact Forces/3(a), Newton-Euler Recursive Inverse Dynamics Block/5(a)
  dd_theta/1 -> Newton-Euler Recursive Inverse Dynamics Block/3(dd_theta)
  Constant9/1 -> Cable Contact Forces/8(eta)
  Constant4/1 -> Cable Contact Forces/6(r_drum)
  theta/1 -> Newton-Euler Recursive Inverse Dynamics Block/1(theta), Cable Contact Forces/2(theta)
  Constant2/1 -> Cable Contact Forces/4(d), Newton-Euler Recursive Inverse Dynamics Block/6(d)
  Constant3/1 -> Cable Contact Forces/5(r), Newton-Euler Recursive Inverse Dynamics Block/7(r)
  Constant10/1 -> Cable Contact Forces/9(mu)
  d_theta/1 -> Newton-Euler Recursive Inverse Dynamics Block/2(d_theta)
  Constant1/1 -> Newton-Euler Recursive Inverse Dynamics Block/4(m)
  Constant5/1 -> Newton-Euler Recursive Inverse Dynamics Block/8(g)
  Newton-Euler Recursive Inverse Dynamics Block/1(u) -> tau/1
  Cable Contact Forces/2(T_ec) -> Newton-Euler Recursive Inverse Dynamics Block/10(T_ec)
  Cable Contact Forces/1(F_ec) -> Newton-Euler Recursive Inverse Dynamics Block/9(F_ec)
  Constant12/1 -> Cable Contact Forces/7(l_link)
  tau_c/1 -> Cable Contact Forces/1(tau_m)

== system Manipulator_Dynamics_testing/Dynamic Model of the arm/M_inv(theta)/Newton-Euler Inverse Dynamics Block 16 ==
  note: Constants
  theta : Inport
  d_theta : Inport  Port=2
  dd_theta : Inport  Port=3
  tau_c : Inport  Port=4
  Cable Contact Forces : MATLAB Function  TreatAsAtomicUnit=on
  Constant : Constant  Value=a
  Constant1 : Constant  Value=m
  Constant10 : Constant  Value=mu_cable
  Constant12 : Constant  Value=l_link
  Constant2 : Constant  Value=d
  Constant3 : Constant  Value=r
  Constant4 : Constant  Value=r_drum
  Constant5 : Constant  Value=g
  Constant9 : Constant  Value=eta
  Newton-Euler Recursive Inverse Dynamics Block : MATLAB Function  TreatAsAtomicUnit=on
  tau : Outport
  wires:
  Constant/1 -> Cable Contact Forces/3(a), Newton-Euler Recursive Inverse Dynamics Block/5(a)
  dd_theta/1 -> Newton-Euler Recursive Inverse Dynamics Block/3(dd_theta)
  Constant9/1 -> Cable Contact Forces/8(eta)
  Constant4/1 -> Cable Contact Forces/6(r_drum)
  theta/1 -> Newton-Euler Recursive Inverse Dynamics Block/1(theta), Cable Contact Forces/2(theta)
  Constant2/1 -> Cable Contact Forces/4(d), Newton-Euler Recursive Inverse Dynamics Block/6(d)
  Constant3/1 -> Cable Contact Forces/5(r), Newton-Euler Recursive Inverse Dynamics Block/7(r)
  Constant10/1 -> Cable Contact Forces/9(mu)
  d_theta/1 -> Newton-Euler Recursive Inverse Dynamics Block/2(d_theta)
  Constant1/1 -> Newton-Euler Recursive Inverse Dynamics Block/4(m)
  Constant5/1 -> Newton-Euler Recursive Inverse Dynamics Block/8(g)
  Newton-Euler Recursive Inverse Dynamics Block/1(u) -> tau/1
  Cable Contact Forces/2(T_ec) -> Newton-Euler Recursive Inverse Dynamics Block/10(T_ec)
  Cable Contact Forces/1(F_ec) -> Newton-Euler Recursive Inverse Dynamics Block/9(F_ec)
  Constant12/1 -> Cable Contact Forces/7(l_link)
  tau_c/1 -> Cable Contact Forces/1(tau_m)

== system Manipulator_Dynamics_testing/Dynamic Model of the arm/M_inv(theta)/Newton-Euler Inverse Dynamics Block 17 ==
  note: Constants
  theta : Inport
  d_theta : Inport  Port=2
  dd_theta : Inport  Port=3
  tau_c : Inport  Port=4
  Cable Contact Forces : MATLAB Function  TreatAsAtomicUnit=on
  Constant : Constant  Value=a
  Constant1 : Constant  Value=m
  Constant10 : Constant  Value=mu_cable
  Constant12 : Constant  Value=l_link
  Constant2 : Constant  Value=d
  Constant3 : Constant  Value=r
  Constant4 : Constant  Value=r_drum
  Constant5 : Constant  Value=g
  Constant9 : Constant  Value=eta
  Newton-Euler Recursive Inverse Dynamics Block : MATLAB Function  TreatAsAtomicUnit=on
  tau : Outport
  wires:
  Constant/1 -> Cable Contact Forces/3(a), Newton-Euler Recursive Inverse Dynamics Block/5(a)
  dd_theta/1 -> Newton-Euler Recursive Inverse Dynamics Block/3(dd_theta)
  Constant9/1 -> Cable Contact Forces/8(eta)
  Constant4/1 -> Cable Contact Forces/6(r_drum)
  theta/1 -> Newton-Euler Recursive Inverse Dynamics Block/1(theta), Cable Contact Forces/2(theta)
  Constant2/1 -> Cable Contact Forces/4(d), Newton-Euler Recursive Inverse Dynamics Block/6(d)
  Constant3/1 -> Cable Contact Forces/5(r), Newton-Euler Recursive Inverse Dynamics Block/7(r)
  Constant10/1 -> Cable Contact Forces/9(mu)
  d_theta/1 -> Newton-Euler Recursive Inverse Dynamics Block/2(d_theta)
  Constant1/1 -> Newton-Euler Recursive Inverse Dynamics Block/4(m)
  Constant5/1 -> Newton-Euler Recursive Inverse Dynamics Block/8(g)
  Newton-Euler Recursive Inverse Dynamics Block/1(u) -> tau/1
  Cable Contact Forces/2(T_ec) -> Newton-Euler Recursive Inverse Dynamics Block/10(T_ec)
  Cable Contact Forces/1(F_ec) -> Newton-Euler Recursive Inverse Dynamics Block/9(F_ec)
  Constant12/1 -> Cable Contact Forces/7(l_link)
  tau_c/1 -> Cable Contact Forces/1(tau_m)

== system Manipulator_Dynamics_testing/Dynamic Model of the arm/M_inv(theta)/Newton-Euler Inverse Dynamics Block 2 ==
  note: Constants
  theta : Inport
  d_theta : Inport  Port=2
  dd_theta : Inport  Port=3
  tau_c : Inport  Port=4
  Cable Contact Forces : MATLAB Function  TreatAsAtomicUnit=on
  Constant : Constant  Value=a
  Constant1 : Constant  Value=m
  Constant10 : Constant  Value=mu_cable
  Constant12 : Constant  Value=l_link
  Constant2 : Constant  Value=d
  Constant3 : Constant  Value=r
  Constant4 : Constant  Value=r_drum
  Constant5 : Constant  Value=g
  Constant9 : Constant  Value=eta
  Newton-Euler Recursive Inverse Dynamics Block : MATLAB Function  TreatAsAtomicUnit=on
  tau : Outport
  wires:
  Constant/1 -> Cable Contact Forces/3(a), Newton-Euler Recursive Inverse Dynamics Block/5(a)
  dd_theta/1 -> Newton-Euler Recursive Inverse Dynamics Block/3(dd_theta)
  Constant9/1 -> Cable Contact Forces/8(eta)
  Constant4/1 -> Cable Contact Forces/6(r_drum)
  theta/1 -> Newton-Euler Recursive Inverse Dynamics Block/1(theta), Cable Contact Forces/2(theta)
  Constant2/1 -> Cable Contact Forces/4(d), Newton-Euler Recursive Inverse Dynamics Block/6(d)
  Constant3/1 -> Cable Contact Forces/5(r), Newton-Euler Recursive Inverse Dynamics Block/7(r)
  Constant10/1 -> Cable Contact Forces/9(mu)
  d_theta/1 -> Newton-Euler Recursive Inverse Dynamics Block/2(d_theta)
  Constant1/1 -> Newton-Euler Recursive Inverse Dynamics Block/4(m)
  Constant5/1 -> Newton-Euler Recursive Inverse Dynamics Block/8(g)
  Newton-Euler Recursive Inverse Dynamics Block/1(u) -> tau/1
  Cable Contact Forces/2(T_ec) -> Newton-Euler Recursive Inverse Dynamics Block/10(T_ec)
  Cable Contact Forces/1(F_ec) -> Newton-Euler Recursive Inverse Dynamics Block/9(F_ec)
  Constant12/1 -> Cable Contact Forces/7(l_link)
  tau_c/1 -> Cable Contact Forces/1(tau_m)

== system Manipulator_Dynamics_testing/Dynamic Model of the arm/M_inv(theta)/Newton-Euler Inverse Dynamics Block 3 ==
  note: Constants
  theta : Inport
  d_theta : Inport  Port=2
  dd_theta : Inport  Port=3
  tau_c : Inport  Port=4
  Cable Contact Forces : MATLAB Function  TreatAsAtomicUnit=on
  Constant : Constant  Value=a
  Constant1 : Constant  Value=m
  Constant10 : Constant  Value=mu_cable
  Constant12 : Constant  Value=l_link
  Constant2 : Constant  Value=d
  Constant3 : Constant  Value=r
  Constant4 : Constant  Value=r_drum
  Constant5 : Constant  Value=g
  Constant9 : Constant  Value=eta
  Newton-Euler Recursive Inverse Dynamics Block : MATLAB Function  TreatAsAtomicUnit=on
  tau : Outport
  wires:
  Constant/1 -> Cable Contact Forces/3(a), Newton-Euler Recursive Inverse Dynamics Block/5(a)
  dd_theta/1 -> Newton-Euler Recursive Inverse Dynamics Block/3(dd_theta)
  Constant9/1 -> Cable Contact Forces/8(eta)
  Constant4/1 -> Cable Contact Forces/6(r_drum)
  theta/1 -> Newton-Euler Recursive Inverse Dynamics Block/1(theta), Cable Contact Forces/2(theta)
  Constant2/1 -> Cable Contact Forces/4(d), Newton-Euler Recursive Inverse Dynamics Block/6(d)
  Constant3/1 -> Cable Contact Forces/5(r), Newton-Euler Recursive Inverse Dynamics Block/7(r)
  Constant10/1 -> Cable Contact Forces/9(mu)
  d_theta/1 -> Newton-Euler Recursive Inverse Dynamics Block/2(d_theta)
  Constant1/1 -> Newton-Euler Recursive Inverse Dynamics Block/4(m)
  Constant5/1 -> Newton-Euler Recursive Inverse Dynamics Block/8(g)
  Newton-Euler Recursive Inverse Dynamics Block/1(u) -> tau/1
  Cable Contact Forces/2(T_ec) -> Newton-Euler Recursive Inverse Dynamics Block/10(T_ec)
  Cable Contact Forces/1(F_ec) -> Newton-Euler Recursive Inverse Dynamics Block/9(F_ec)
  Constant12/1 -> Cable Contact Forces/7(l_link)
  tau_c/1 -> Cable Contact Forces/1(tau_m)

== system Manipulator_Dynamics_testing/Dynamic Model of the arm/M_inv(theta)/Newton-Euler Inverse Dynamics Block 4 ==
  note: Constants
  theta : Inport
  d_theta : Inport  Port=2
  dd_theta : Inport  Port=3
  tau_c : Inport  Port=4
  Cable Contact Forces : MATLAB Function  TreatAsAtomicUnit=on
  Constant : Constant  Value=a
  Constant1 : Constant  Value=m
  Constant10 : Constant  Value=mu_cable
  Constant12 : Constant  Value=l_link
  Constant2 : Constant  Value=d
  Constant3 : Constant  Value=r
  Constant4 : Constant  Value=r_drum
  Constant5 : Constant  Value=g
  Constant9 : Constant  Value=eta
  Newton-Euler Recursive Inverse Dynamics Block : MATLAB Function  TreatAsAtomicUnit=on
  tau : Outport
  wires:
  Constant/1 -> Cable Contact Forces/3(a), Newton-Euler Recursive Inverse Dynamics Block/5(a)
  dd_theta/1 -> Newton-Euler Recursive Inverse Dynamics Block/3(dd_theta)
  Constant9/1 -> Cable Contact Forces/8(eta)
  Constant4/1 -> Cable Contact Forces/6(r_drum)
  theta/1 -> Newton-Euler Recursive Inverse Dynamics Block/1(theta), Cable Contact Forces/2(theta)
  Constant2/1 -> Cable Contact Forces/4(d), Newton-Euler Recursive Inverse Dynamics Block/6(d)
  Constant3/1 -> Cable Contact Forces/5(r), Newton-Euler Recursive Inverse Dynamics Block/7(r)
  Constant10/1 -> Cable Contact Forces/9(mu)
  d_theta/1 -> Newton-Euler Recursive Inverse Dynamics Block/2(d_theta)
  Constant1/1 -> Newton-Euler Recursive Inverse Dynamics Block/4(m)
  Constant5/1 -> Newton-Euler Recursive Inverse Dynamics Block/8(g)
  Newton-Euler Recursive Inverse Dynamics Block/1(u) -> tau/1
  Cable Contact Forces/2(T_ec) -> Newton-Euler Recursive Inverse Dynamics Block/10(T_ec)
  Cable Contact Forces/1(F_ec) -> Newton-Euler Recursive Inverse Dynamics Block/9(F_ec)
  Constant12/1 -> Cable Contact Forces/7(l_link)
  tau_c/1 -> Cable Contact Forces/1(tau_m)
